simulink model "BLDC_Data_Gen"  (R2024b)
settings: Solver=VariableStepAuto  StartTime=0.0  StopTime=10.0  RelTol=1e-3
undefined symbols (not defined in the file): dspblkCoreblockFVToolHelper, gcbh
settings Model: Creator=Aayushman Naik  LastModifiedBy=Aayushman Naik

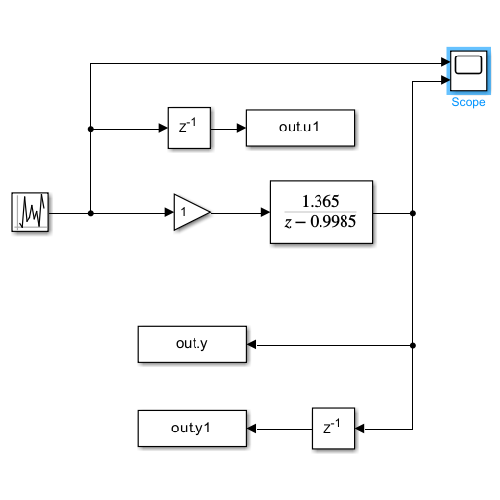
[thumbnail: Simulink's stored preview of the top-level diagram]
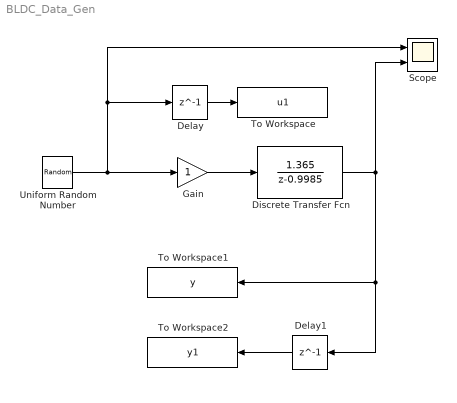
== system BLDC_Data_Gen ==
  Delay : Delay  DelayLength=1
  Delay1 : Delay  DelayLength=1
  Discrete Transfer Fcn : DiscreteTransferFcn  LoadFcn=dspblkCoreblockFVToolHelper(gcbh,'load');  Numerator=[1.365]  Denominator=[1 -0.9985]
      settings: CopyFcn=dspblkCoreblockFVToolHelper(gcbh,'copy');  DeleteFcn=dspblkCoreblockFVToolHelper(gcbh,'close');  ModelCloseFcn=dspblkCoreblockFVToolHelper(gcbh,'close');  PreSaveFcn=dspblkCoreblockFVToolHelper(gcbh,'presave');  PostSaveFcn=dspblkCoreblockFVToolHelper(gcbh,'postsave');  CloseFcn=dspblkCoreblockFVToolHelper(gcbh,'close');
  Gain : Gain
  Scope : Scope  NumInputPorts=2
  To Workspace : ToWorkspace  VariableName=u1  SaveFormat=Timeseries  SampleTime=-1
  To Workspace1 : ToWorkspace  VariableName=y  SaveFormat=Timeseries  SampleTime=-1
  To Workspace2 : ToWorkspace  VariableName=y1  SaveFormat=Timeseries  SampleTime=-1
  Uniform Random Number : UniformRandomNumber  SampleTime=0.1
  wires:
  Uniform Random Number/1 -> Scope/1, Delay/1, Gain/1
  Gain/1 -> Discrete Transfer Fcn/1
  Delay/1 -> To Workspace/1
  Discrete Transfer Fcn/1 -> Delay1/1, To Workspace1/1, Scope/2
  Delay1/1 -> To Workspace2/1
